simulink model "rosHelper"  (R2024b)
settings: Solver=FixedStepAuto  StartTime=0.0  StopTime=50  RelTol=1e-3
model workspace (MAT data in the model file):
  SL_Bus_ROSEnable64bitIntegers = 1
  SL_ROS_VariableLengthArrays_MaxSizes.CommonInfo.ArrayTruncateAction = 'EmitWarning'
  SL_ROS_VariableLengthArrays_MaxSizes.MsgTypeMap = containers.Map
  SL_ROS_VariableLengthArrays_MaxSizes.MsgTypeMap.serialization.keys = {'std_msgs/Float32MultiArray', 'std_msgs/Float64MultiArray'}
  SL_ROS_VariableLengthArrays_MaxSizes.MsgTypeMap.serialization.values{1}.PropertyName = 'data'
  SL_ROS_VariableLengthArrays_MaxSizes.MsgTypeMap.serialization.values{1}.DataType = 'single'
  SL_ROS_VariableLengthArrays_MaxSizes.MsgTypeMap.serialization.values{1}.MaxLength = 10000
  SL_ROS_VariableLengthArrays_MaxSizes.MsgTypeMap.serialization.values{2}.PropertyName = 'data'
  SL_ROS_VariableLengthArrays_MaxSizes.MsgTypeMap.serialization.values{2}.DataType = 'double'
  SL_ROS_VariableLengthArrays_MaxSizes.MsgTypeMap.serialization.values{2}.MaxLength = 10000
  SL_ROS_VariableLengthArrays_MaxSizes.MsgTypeMap.serialization.uniformity = 0
  SL_ROS_VariableLengthArrays_MaxSizes.MsgTypeMap.serialization.keyType = 'char'
  SL_ROS_VariableLengthArrays_MaxSizes.MsgTypeMap.serialization.valueType = 'any'
libraries: roshelperlib x15
settings Model: DataDictionary=ros2lib.sldd  Creator=cstabile  LastModifiedBy=jbrault
settings SolverCC: DateTimeAtSimulationTimeZero=[]
settings OptimizationCC: EnhancedBackFolding=on  PassReuseOutputArgsAs=Individual arguments  ZeroExternalMemoryAtStartup=off  ZeroInternalMemoryAtStartup=off  MaxStackSize=64  OptimizeBlockOrder=speed  DifferentSizesBufferReuse=on  OptimizationCustomize=off  EfficientTunableParamExpr=on
settings DebuggingCC: ParameterTunabilityLossMsg=error
settings RTWCC: Description=Embedded Coder  SystemTargetFile=ert.tlc  HardwareBoard=Robot Operating System 2 (ROS 2)  TLCOptions="-aInlineSetEventsForThisBaseRateFcn=TLC_FALSE -aSuppressMultiTaskScheduler=TLC_FALSE  -aRateBasedStepFcn=0"  TemplateMakefile=ert_default_tmf  Toolchain=Colcon Tools  TargetLang=C++
settings CodeAppCC: ForceParamTrailComments=on  IgnoreCustomStorageClasses=off  OperatorAnnotations=on  SimulinkDataObjDesc=on  SFDataObjDesc=on  InsertBlockDesc=on
settings ERTTargetCC: CodeInterfacePackaging=C++ class  InlinedParameterPlacement=Hierarchical  RootIOFormat=Structure reference  DynamicArrayContainerType=coder::array

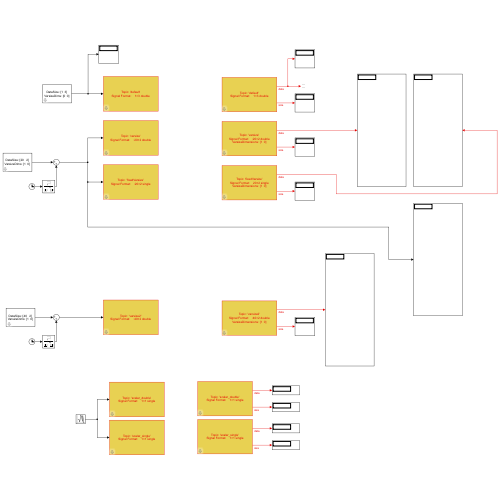
[thumbnail: Simulink's stored preview of the top-level diagram]
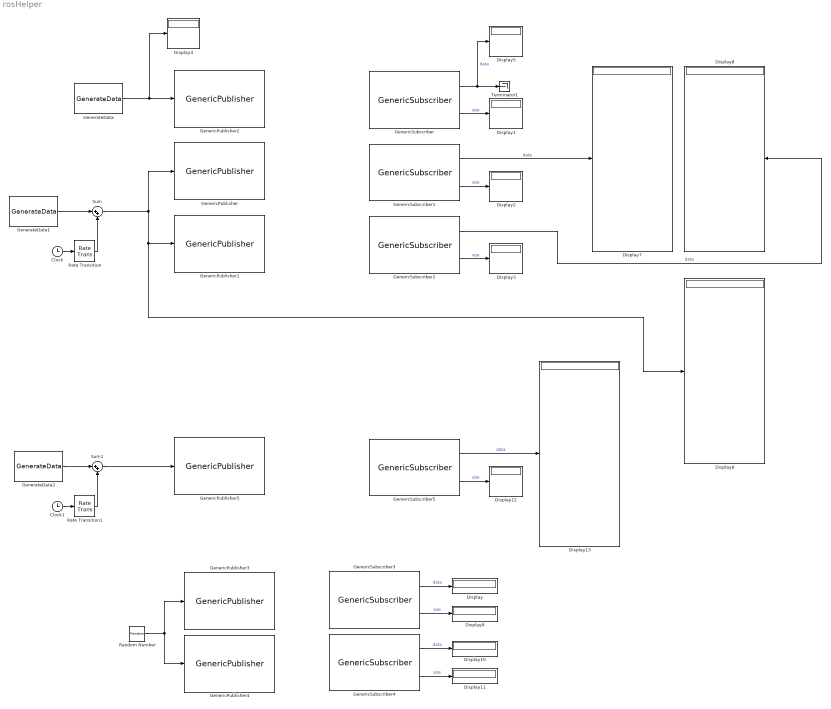
== system rosHelper ==
  Clock : Clock
  Clock1 : Clock
  Display{,1..13} (14 alike) : Display
  GenerateData : roshelperlib/GenerateData  dataSize=[1 3]  varsizeDims=[]
  GenerateData1 : roshelperlib/GenerateData  dataSize=[20 2]  varsizeDims=[1 0]
  GenerateData2 : roshelperlib/GenerateData  dataSize=[40 2]  varsizeDims=[1 0]
  GenericPublisher : roshelperlib/GenericPublisher  userDataType=double  dims=[20 2]  topicName='varsize'  isVarsize=on  varsizeDims=[1 0]
  GenericPublisher1 : roshelperlib/GenericPublisher  userDataType=single  dims=[20 2]  topicName='fixedVarsize'  isVarsize=on  varsizeDims=[1 0]
  GenericPublisher2 : roshelperlib/GenericPublisher  userDataType=double  dims=[1 3]  topicName='default'  isVarsize=off  varsizeDims=[1 1]
  GenericPublisher3 : roshelperlib/GenericPublisher  userDataType=single  dims=[1 1]  topicName='scalar_double'  isVarsize=off  varsizeDims=[1 0]
  GenericPublisher4 : roshelperlib/GenericPublisher  userDataType=single  dims=[1 1]  topicName='scalar_single'  isVarsize=off  varsizeDims=[1 0]
  GenericPublisher5 : roshelperlib/GenericPublisher  userDataType=double  dims=[40 2]  topicName='varsize2'  isVarsize=on  varsizeDims=[1 0]
  GenericSubscriber : roshelperlib/GenericSubscriber  userDataType=double  dims=[1 3]  topicName='default'  isVarsize=off  varsizeDims=[]  returnFixedTF=off
  GenericSubscriber1 : roshelperlib/GenericSubscriber  userDataType=double  dims=[20 2]  topicName='varsize'  isVarsize=on  varsizeDims=[1 0]  returnFixedTF=off
  GenericSubscriber2 : roshelperlib/GenericSubscriber  userDataType=single  dims=[20 2]  topicName='fixedVarsize'  isVarsize=on  varsizeDims=[1 0]  returnFixedTF=on
  GenericSubscriber3 : roshelperlib/GenericSubscriber  userDataType=single  dims=[1 1]  topicName='scalar_double'  isVarsize=off  varsizeDims=[1 0]  returnFixedTF=off
  GenericSubscriber4 : roshelperlib/GenericSubscriber  userDataType=single  dims=[1 1]  topicName='scalar_single'  isVarsize=off  varsizeDims=[1 0]  returnFixedTF=off
  GenericSubscriber5 : roshelperlib/GenericSubscriber  userDataType=double  dims=[40 2]  topicName='varsize2'  isVarsize=on  varsizeDims=[1 0]  returnFixedTF=off
  Random Number : RandomNumber  SampleTime=0.1
  Rate Transition : RateTransition
  Rate Transition1 : RateTransition
  Sum : Sum  Inputs=|++
  Sum1 : Sum  Inputs=|++
  Terminator1 : Terminator
  wires:
  GenericSubscriber/1 -> Terminator1/1, Display5/1  "data"
  GenericSubscriber/2 -> Display1/1  "size"
  GenericSubscriber1/2 -> Display2/1  "size"
  GenericSubscriber1/1 -> Display7/1  "data"
  GenericSubscriber2/2 -> Display3/1  "size"
  GenericSubscriber2/1 -> Display8/1  "data"
  GenerateData/1 -> Display4/1, GenericPublisher2/1
  Sum/1 -> Display6/1, GenericPublisher1/1, GenericPublisher/1
  GenerateData1/1 -> Sum/1
  Clock/1 -> Rate Transition/1
  Rate Transition/1 -> Sum/2
  Random Number/1 -> GenericPublisher4/1, GenericPublisher3/1
  GenericSubscriber3/1 -> Display/1  "data"
  GenericSubscriber3/2 -> Display9/1  "size"
  GenericSubscriber4/2 -> Display11/1  "size"
  GenericSubscriber4/1 -> Display10/1  "data"
  Rate Transition1/1 -> Sum1/2
  Clock1/1 -> Rate Transition1/1
  GenerateData2/1 -> Sum1/1
  Sum1/1 -> GenericPublisher5/1
  GenericSubscriber5/1 -> Display13/1  "data"
  GenericSubscriber5/2 -> Display12/1  "size"
